simulink model "rtlsdr_QPSK_ascii_message"  (R2021a)
settings: Solver=FixedStepDiscrete  StartTime=0.0  StopTime=60  RelTol=1e-3
PreLoadFcn:
  | %%%%%%%%%%%%%%%%%%%%%%%%%%%%%%%%%%%%%%%%%%%%%%%%%%%%%%%%%%%%%%%%%%%%%%%%%%%
  | % check to see if Simulink library folder is missing from the MATLAB path %
  | %%%%%%%%%%%%%%%%%%%%%%%%%%%%%%%%%%%%%%%%%%%%%%%%%%%%%%%%%%%%%%%%%%%%%%%%%%%
  | if isempty(strfind(path, 'rtlsdr_book_library'))
  | 
  |     % create error window
  |     fig_error = figure(...
  |         'Name', 'Error: RTL-SDR Book Library',...
  |         'Toolbar','none',...
  |         'MenuBar','none',...
  |         'NumberTitle','off',...
  |         'Resize','off',...
  |         'WindowStyle','modal');
  |     fig_error.Position(3) = 600;
  |     fig_error.Position(4) = 150;
  |     fig_axes = axes(...
  |         'Parent',fig_error,...
  |         'Position',[0,0,1,1],...
  |         'visible','off');
  |     % error message
  |     t_title = text(.05,.8,...
  |         'MISSING DIRECTORIES',...
  |         'FontSize',11.5);
  |     t_body = text(.075,.6,...
  |         [{'Simulink cannot find the  \it{<root>}\rm / \it{rtlsdr\_book\_library}\rm  folder in the \it{MATLAB Path}\rm.'},...
  |         {'Please set the MATLAB path following the instructions given in Exercise 2.4.'}],...
  |         'FontSize',10.5);
  |     % buttons
  |     btn_path = uicontrol(...
  |         'Parent',fig_error,...
  |         'String','Set Path Now',...
  |         'FontSize',10,...
  |         'Callback', 'pathtool; close(fig_error);',...
  |         'Position', [fig_error.Position(3)/2-210, 30, 200, 30]);
  |     btn_abort = uicontrol(...
  |         'Parent',fig_error,...
  |         'String','No thanks',...
  |         'FontSize',10,...
  |         'Callback', 'close(fig_error); abort=1;',...
  |         'Position', [fig_error.Position(3)/2+10, 30, 200, 30]);
  | 
  |     % pause to allow user to interact with error box
  |     uiwait(fig_error);
  | 
  |     % abort simulation
  |     try
  |         if abort==1
  |             set_param(gcs, 'SimulationCommand', 'stop');
  |         end
  |     end
  | 
  |     % if user has set path, allow diagram to be updated
  |     if ~exist('abort','var')
  |         % create error window
  |         fig_update = figure(...
  |             'Name', 'Update Diagram',...
  |             'Toolbar','none',...
  |             'MenuBar','none',...
  |             'NumberTitle','off',...
  |             'Resize','off');
  |         fig_update.Position(3) = 400;
  |         fig_update.Position(4) = 120;
  |         fig_axes = axes(...
  |             'Parent',fig_update,...
  |             'Position',[0,0,1,1],...
  |             'visible','off');
  |         % instruction message
  |         t_body = text(.075,.7,...
  |             'Once you have set the path, update the block diagram',...
  |             'FontSize',10.5);
  |         % button
  |         btn_update = uicontrol(...
  |             'Parent',fig_update,...
  |             'String','Update Block Diagram',...
  |             'FontSize',10,...
  |             'Callback', 'set_param(gcs,''SimulationCommand'',''update''); close(gcf)',...
  |             'Position', [fig_update.Position(3)/2-100, 30, 200, 30]);
  |     end
  | 
  |     % clear error components
  |     clear('fig_error','fig_update','fig_axes','t_title','t_body','btn_path','btn_abort','btn_update','abort');
  | 
  | end
  | %%%%%%%%%%%%%%%%%%%%%%%%%%%%%%%%%%%%%%%%%%%%%%%%%%%%%%%%%%%%%%%%%%%%%%%%%%%
  | 
  | 
  | 
  | % ---------------- system parameters ------------------
  | 
  | fs_Tx = 240e3;                           % sampling rate used in the transmitter
  | samp = 50000 - 1;                      % stop time (number of samples in the simulation - 1)
  | fc = 7.5e3;                                  % carrier frequency (IF modulated)
  | Rdata = 2e3;                               % slow data rate chosen for real time demonstration
  | Rsymbol = Rdata/2;                     % QPSK, so 2 samples per symbol
  | fs_Rx = 240e3;                            % sampling rate in the receiver
  | RxDec1 = 5;                                 % decimation at input of Receiver
  | RxDec2 = 6;                                % decimation prior to Coarse Synch
  | RxInt = 3;                                   % interpolation prior to timing and freq synch (output of coarse)
  | OSR = (fs_Rx*RxInt/(RxDec1*RxDec2))/Rsymbol;     % oversampling ratio used in timing and frequency synch
  | 
  | % ---------------- synch loop design ------------------
  | 
  | d = 0.707;                         % damping ratio (using the same for both loops)
  | 
  | % *** CARRIER synch loop *** (note this operates at symbol rate)
  | 
  | T = 1/Rsymbol;                  % sample period
  | Kp = 1;                              % phase detector S-curve is linear
  | Bn = 0.04*Rsymbol;           % bandwidth in Hz
  | Ko = 1;                              % gain of NCO
  | 
  | % calculate the loop filter coefficients for the carrier synch loop
  | K1 = (4*d*Bn*T)/(Ko*Kp*(d+1/(4*d)));
  | K2 = (4*(Bn*T)^2)/(Ko*Kp*(d+1/4*d)^2);
  | 
  | 
  | % *** SYMBOL TIMING synch loop ***
  | 
  | Ts = 1/Rsymbol;                 % symbol period
  | Ks = 3.24;                            % phase detector coefficient
  | BnS = 0.04*Rsymbol;         %  bandwidth in Hz
  | Kn   = 1;                            % gain of numerically controlled clock
  | 
  | % calculate loop filter coefficients
  | Ka = (4*d*BnS*Ts)/(Kn*Ks*(d+1/(4*d)));
  | Kb = (4*(BnS*Ts)^2)/(Kn*Ks*(d+1/4*d)^2);
  | 
  | %------------ design of multirate filter objects ----------
  | 
  | Hd1 = dsp.FIRDecimator(RxDec1,designMultirateFIR(1,RxDec1));            % first stage decimation
  | Hd2 = dsp.FIRDecimator(RxDec2,designMultirateFIR(1,RxDec2));            % second stage decimation
  | Hdf = dsp.FIRDecimator(24,designMultirateFIR(1,24));                           % final stage decimation
  | 
  | Hi = dsp.FIRInterpolator(RxInt,designMultirateFIR(RxInt,1));                   % interpolation
undefined symbols (not defined in the file): rec, src
libraries: simulink_need_slupdate x6, rtlsdr_book_library x5, simulink x4, dspmlti4 x3, dspmtrx3 x3, commdigbbndpm3 x2, commrfcorlib x1, dspbuff3 x1, commutil2 x1, sdrrlib x1, commfilt2 x1
CloseFcn:
  | closefcn_model;
Description:
  | Software, Simulation Examples and Design Exercises Licence Agreement
  | 
  | This license agreement refers to the simulation examples, design exercises and files,
  | and associated software MATLAB and Simulink resources that accompany the book:
  | 
  |      Title: Software Defined Radio using MATLAB & Simulink and the RTL-SDR
  |      Published by Strathclyde Academic Media, 2015
  |      Authored by Robert W. Stewart, Kenneth W. Barlee, Dale S.W. Atkinson,
  |      and Louise H. Crockett
  | 
  | and made available as a download from, www.desktopSDR.com or variously acquired
  | by other means such as via USB storage, cloud storage, disk or any other electronic
  | or optical or magnetic storage mechanism. These files and associated software may
  | be used subject to the terms of agreement of the conditions below:
  | 
  |     Copyright © 2015 Robert W. Stewart, Kenneth W. Barlee, Dale S.W. Atkinson,
  |     and Louise H. Crockett
  |     All rights reserved.
  | 
  | Redistribution and use in source and binary forms, with or without modification, are
  | permitted provided that the following conditions are met:
  | 
  |    1.  Redistributions of source code must retain the above copyright notice, this list of
  |         conditions and the following disclaimer.
  | 
  |    2.  Redistributions in binary form must reproduce the above copyright notice, this
  |         list of conditions and the following disclaimer in the documentation and/or other
  |         materials provided with the distribution.
  | 
  |    3.  Neither the name of the copyright holder nor the names of its contributors may
  |         be used to endorse or promote products derived from this software without
  |         specific prior written permission.
  | 
  |    4.  In all cases, the software is, and all modifications and derivatives of the
  |         software shall be, licensed to you solely for use in conjunction with The
  |         MathWorks, Inc. products and service offerings.
  | 
  | THIS SOFTWARE IS PROVIDED BY THE COPYRIGHT HOLDERS AND CONTRIBUTORS
  | "AS IS" AND ANY EXPRESS OR IMPLIED WARRANTIES, INCLUDING, BUT NOT LIMITED
  | TO, THE IMPLIED WARRANTIES OF MERCHANTABILITY AND FITNESS FOR A
  | PARTICULAR PURPOSE ARE DISCLAIMED. IN NO EVENT SHALL THE COPYRIGHT
  | HOLDER OR CONTRIBUTORS BE LIABLE FOR ANY DIRECT, INDIRECT, INCIDENTAL,
  | SPECIAL, EXEMPLARY, OR CONSEQUENTIAL DAMAGES (INCLUDING, BUT NOT
  | LIMITED TO, PROCUREMENT OF SUBSTITUTE GOODS OR SERVICES; LOSS OF USE,
  | DATA, OR PROFITS; OR BUSINESS INTERRUPTION) HOWEVER CAUSED AND ON ANY
  | THEORY OF LIABILITY, WHETHER IN CONTRACT, STRICT LIABILITY, OR TORT
  | (INCLUDING NEGLIGENCE OR OTHERWISE) ARISING IN ANY WAY OUT OF THE USE
  | OF THIS SOFTWARE, EVEN IF ADVISED OF THE POSSIBILITY OF SUCH DAMAGE.
  | 
  | 
  | Audio Tracks used in Simulations Examples and Design Exercises
  | 
  | The music and vocal files used within the Examples files and software within the book
  | were variously written, arranged, performed, recorded and produced by Garrey Rice,
  | Adam Struth, Jamie Struth, Iain Thistlethwaite and also Marshall Craigmyle who
  | collectively, and individually where appropriate, assert and retain all of their copyright,
  | performance and artistic rights. Permission to use and reproduce this music is
  | granted for all purposes associated with MATLAB and Simulink software and the
  | simulation examples and design exercises files that accompany this book. Requests to
  | use the music for any other purpose should be directed to: info@desktopSDR.com.
  | For information on music track names, full credits, and links to the musicians please
  | refer to www.desktopSDR.com/more/audio.
settings Model: ModifiedByFormat=desktopSDR Team  SimulationMode=accelerator  Creator=desktopSDR Team  LastModifiedBy=desktopSDR Team
settings SolverCC: AlgebraicLoopSolver=TrustRegion
settings DataIOCC: SaveFormat=Array  SaveOutput=off  SignalLogging=off  SaveTime=off  ReturnWorkspaceOutputs=off
settings OptimizationCC: EfficientMapNaN2IntZero=off  LifeSpan=inf
settings DebuggingCC: UnderspecifiedInitializationDetection=Classic  MergeDetectMultiDrivingBlocksExec=none  SolverPrmCheckMsg=warning  ParameterPrecisionLossMsg=none  AllowSymbolicDim=off  SFUnexpectedBacktrackingDiag=warning  SFNoUnconditionalDefaultTransitionDiag=warning  SFExecutionAtInitializationDiag=none  SFMachineParentedDataDiag=warning  ArithmeticOperatorsInVariantConditions=warning
settings HardwareCC: ProdBitPerPointer=32  ProdBitPerSizeT=32  ProdBitPerPtrDiffT=32  ProdLargestAtomicFloat=None  ProdIntDivRoundTo=Undefined  ProdEndianess=Unspecified  ProdWordSize=32  ProdHWDeviceType=32-bit Generic  TargetBitPerPointer=64  TargetBitPerSizeT=64  TargetBitPerPtrDiffT=64  TargetLongLongMode=on  TargetIntDivRoundTo=Zero  TargetEndianess=LittleEndian  TargetWordSize=64  TargetHWDeviceType=MATLAB Host  ProdEqTarget=off
settings ModelReferenceCC: PropagateSignalLabelsOutOfModel=off
settings SFSimCC: SimUseLocalCustomCode=off  CustomCodeUndefinedFunction=UseInterfaceOnly
settings RTWCC: RTWUseLocalCustomCode=off
settings CodeAppCC: MaxIdLength=128  StateflowObjectComments=on
settings GRTTargetCC: TargetLangStandard=C89/C90 (ANSI)  CombineOutputUpdateFcns=off  GRTInterface=on
settings ConfigComp: CovMetricSettings=dw  CovSaveCumulativeToWorkspaceVar=on  CovSaveSingleToWorkspaceVar=on  CovExternalEMLEnable=off  CovSFcnEnable=off

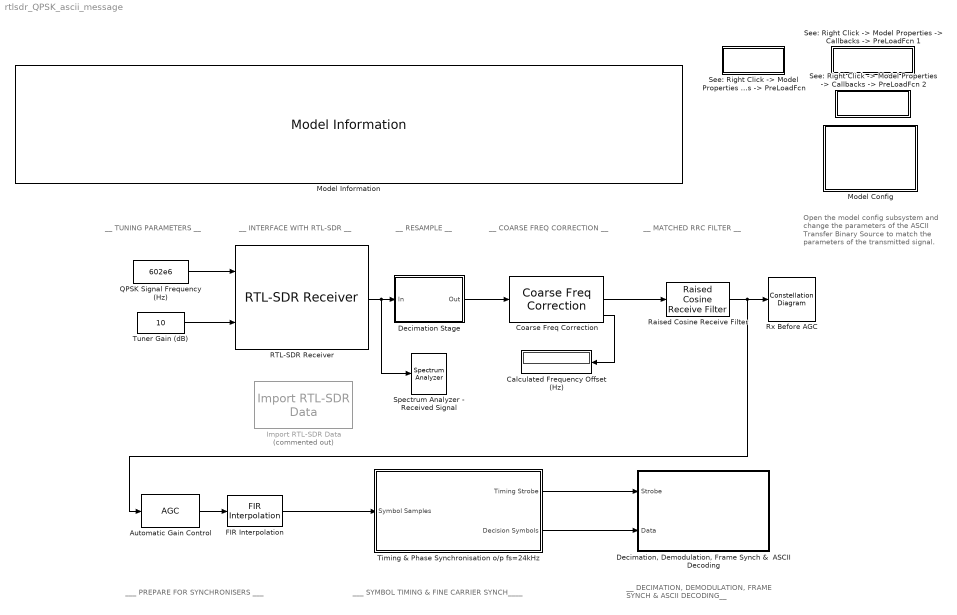
== system rtlsdr_QPSK_ascii_message ==
  note: ___ PREPARE FOR SYNCHRONISERS ___
  note: ___ SYMBOL TIMING & FINE CARRIER SYNCH____
  note: __ DECIMATION, DEMODULATION,
      | FRAME SYNCH & ASCII DECODING__
  note: __ TUNING PARAMETERS __
  note: __ INTERFACE WITH RTL-SDR __
  note: __ RESAMPLE __
  note: __ MATCHED RRC FILTER __
  note: __ COARSE FREQ CORRECTION __
  note: Open the model config subsystem and change the parameters of the ASCII Transfer Binary Source to match the parameters of the transmitted signal.
  Automatic Gain Control : commrfcorlib/AGC  LegacyMode=off  DetectorMethod=Rectifier  LoopMethod=Linear  UpdatePeriod=128  StepSize=0.05  AdaptationStepSize=(0.05)/(128)  DesiredOutputPower=1  AveragingLength=128  MaximumGain=20  MaxPowerGain=20  GainOutputPort=off  InputPowerOutputPort=off  SimulateUsing=Code generation
  Calculated Frequency Offset (Hz) : Display
  Coarse Freq Correction : rtlsdr_book_library/Sync Tools for Digital Comms/Coarse Freq Correction  frm_size=4096
      settings: SourceProductName=RTL-SDR Book Library
  Decimation Stage : Subsystem
      mask Display: disp('Decimation');
  "Decimation, Demodulation, Frame Synch &  ASCII Decoding" : Subsystem  mask(Receiver Parameter Settings){msg_len=rec.msg_len, fs=src.fs, ascii_len=8}
      mask prompts: msg_len "Message Length (chars):"; fs "Sampling Frequency:"; ascii_len "ACSII Length:"
      mask help: This subsystem decimates the signal back to symbol rate by storing only the valid samples that are chosen using the 'strobe' input. It then demodulates the samples back to bits to perform frame synchronisation and finally ASCII decoding. The parameters should match those set in the transmitter for the process to be successful.
      mask Callback msg_len: ASCII_receive_mtchd_filt;
      mask Callback fs: ASCII_receive_mtchd_filt;
      mask Callback ascii_len: ASCII_receive_mtchd_filt;
  FIR Interpolation : dspmlti4/FIR Interpolation  FilterSource=Filter object  PrivateCoeffs=0  h=fir1(71,1/RxInt)  L=RxInt  FilterObject=Hi  InputProcessing=Columns as channels (frame based)  framing=Allow multirate processing  outputBufInitCond=0  roundingMode=Floor  overflowMode=off  firstCoeffDataTypeStr=Inherit: Same word length as input  firstCoeffMin=[]  firstCoeffMax=[]  firstCoeffLastDataTypeStr=Inherit: Same word length as input  outputDataTypeStr=Inherit: Same as accumulator  outputMin=[]  outputMax=[]  outputLastDataTypeStr=Inherit: Same as accumulator
  Import RTL-SDR Data : rtlsdr_book_library/Additional Tools/Import RTL-SDR Data  Commented=on  filename=rec_data\qpsk_ascii_msg.mat  frm_size=4096  data_type=single
      settings: SourceProductName=RTL-SDR Book Library
  Model Config : Subsystem
      mask Display: disp('Model\nConfig')
  Model Information : rtlsdr_book_library/Additional Tools/Model Information/Model Information
      settings: SourceProductName=RTL-SDR Book Library
  "QPSK Signal Frequency (Hz) " : Constant  Value=602e6
  RTL-SDR Receiver : sdrrlib/RTL-SDR Receiver  IPAddress=0  CenterFrequencySource=Input port  CenterFrequency=433.9e6  GainSource=Input port  Gain=15  ADCRate=240e3  FrequencyCorrection=0  LostSamplesOutputPort=off  LatencyOutputPort=off  OutputDataType=single  FrameLength=4096  EnableBurstMode=off  NumFramesInBurst=20  sobjType=sdrr.internal.SDRRTLReceiverSL  dataUDPPort=-1  ctrlUDPPort=-1  subDeviceList=nosubdev  sdrBlockType=SDRBlockTypeSLT.SDRRxBlock  requester=UNUSED_BY_SFCN  sdrExecutionMode=SDRExecutionModeSLT.ExecModeHW  BypassUserLogic=off  DecimatorSelect=DDC decimator  SourceSelect=RF data  SineAmplitude=16000  EnableInternalClock=off  BypassIQBalance=off  IFBandwidth=40e6  ADCRateSource=Dialog  IntermediateFrequency=0  DecimationFactorSource=Dialog  DecimationFactor=512  RFFrequencyIsTunable=logical(1)  SampleTime=(4096)/(240e3)  IFBandwidthSource=Dialog  SineFrequency=30000  BypassDCBlockingFilter=off  IntermediateFrequencySource=Dialog  IQBalanceCoefficients=64  SkipAllHardwareResetAndInitialization=off  EnableIQCalibrationTable=on  CacheIQCalibrationTable=off  EnableOffsetTuning=off  EnableRTLAGC=off  EnableTestMode=off  EnableTunerAGC=off  FrequencyCorrectionSource=Dialog  NumMLBuffers=128  NumUSBBuffers=16  RTLCrystalFrequency=28800000  TunerCrystalFrequency=28800000
      settings: SourceProductBaseCode=RTLSDR
  Raised Cosine Receive Filter : commfilt2/Raised Cosine Receive Filter  filtType=Square root  R=0.5  filtSpan=12  N=fs_Rx/(RxDec1*RxDec2*Rsymbol)  downFactor=1  downOffset=0  filterGain=1  InputProcessing=Columns as channels (frame based)  RateOptions=Enforce single-rate processing  framing=Allow multirate processing  checkCoeff=off  variableName=rcRxFilt1  currentFiltSpan=12  D=(12)/2  inputOffset=0  sampMode=Mute  saveAsFlag=0  rateMode=Downsampling  checkGain=Normalized  launchFVT=on  roundingMode=Floor  overflowMode=off  coeffDataTypeStr=Inherit: Same word length as input  coeffMin=[]  coeffMax=[]  coeffLastDataTypeStr=Inherit: Same word length as input  accumDataTypeStr=Inherit: Same as product output  accumLastDataTypeStr=Inherit: Same as product output  outputDataTypeStr=Inherit: Same as accumulator  outputMin=[]  outputMax=[]  outputLastDataTypeStr=Inherit: Same as accumulator
  Rx Before AGC : ConstellationDiagram
  "See: Right Click -> Model Properties -> Callbacks -> PreLoadFcn" : Subsystem
      mask Display:
      | OSR = evalin('base', 'OSR');
      | fprintf(['OSR = ',num2str(OSR)]);
  "See: Right Click -> Model Properties -> Callbacks -> PreLoadFcn 1" : Subsystem
      mask Display:
      | Rsymbol = evalin('base', 'Rsymbol');
      | fprintf(['Rsymbol = ',num2str(Rsymbol/1e3),' ksps']);
  "See: Right Click -> Model Properties -> Callbacks -> PreLoadFcn 2" : Subsystem
      mask Display:
      | fs_Rx = evalin('base', 'fs_Rx');
      | fprintf(['fs_Rx = ',num2str(fs_Rx/1e3),' kHz']);
  Spectrum Analyzer - Received Signal : SpectrumAnalyzer
  Timing & Phase Synchronisation o/p fs=24kHz : Subsystem
  Tuner Gain (dB) : Constant  Value=10
  wires:
  Raised Cosine Receive Filter/1 -> Rx Before AGC/1, Automatic Gain Control/1
  Automatic Gain Control/1 -> FIR Interpolation/1
  Tuner Gain (dB)/1 -> RTL-SDR Receiver/2
  "QPSK Signal Frequency (Hz) "/1 -> RTL-SDR Receiver/1
  Coarse Freq Correction/2 -> Raised Cosine Receive Filter/1
  FIR Interpolation/1 -> Timing & Phase Synchronisation o/p fs=24kHz/1(Symbol Samples)
  Timing & Phase Synchronisation o/p fs=24kHz/2(Decision Symbols) -> "Decimation, Demodulation, Frame Synch &  ASCII Decoding"/2(Data)
  Decimation Stage/1(Out) -> Coarse Freq Correction/1
  Coarse Freq Correction/3 -> Calculated Frequency Offset (Hz)/1
  Timing & Phase Synchronisation o/p fs=24kHz/1(Timing Strobe) -> "Decimation, Demodulation, Frame Synch &  ASCII Decoding"/1(Strobe)
  RTL-SDR Receiver/1 -> Spectrum Analyzer - Received Signal/1, Decimation Stage/1(In)

== system rtlsdr_QPSK_ascii_message/Decimation Stage ==
  In : Inport
  FIR Decimation x5 o/p fs=48kHz : dspmlti4/FIR Decimation  FilterSource=Filter object  h=fir1(35,1/5)  D=5  filtStruct=Direct form  FilterObject=Hd1  InputProcessing=Columns as channels (frame based)  framing=Allow multirate processing  inputOffset=0  outputBufInitCond=0  roundingMode=Floor  overflowMode=off  firstCoeffDataTypeStr=Inherit: Same word length as input  firstCoeffMin=[]  firstCoeffMax=[]  firstCoeffLastDataTypeStr=Inherit: Same word length as input  outputDataTypeStr=Inherit: Same as accumulator  outputMin=[]  outputMax=[]  outputLastDataTypeStr=Inherit: Same as accumulator
  "FIR Decimation x6 o/p fs=8kHz " : dspmlti4/FIR Decimation  FilterSource=Filter object  h=fir1(75,1/6)  D=6  filtStruct=Direct form  FilterObject=Hd2  InputProcessing=Columns as channels (frame based)  framing=Allow multirate processing  inputOffset=0  outputBufInitCond=0  roundingMode=Floor  overflowMode=off  firstCoeffDataTypeStr=Inherit: Same word length as input  firstCoeffMin=[]  firstCoeffMax=[]  firstCoeffLastDataTypeStr=Inherit: Same word length as input  outputDataTypeStr=Inherit: Same as accumulator  outputMin=[]  outputMax=[]  outputLastDataTypeStr=Inherit: Same as accumulator
  Out : Outport
  wires:
  "FIR Decimation x6 o/p fs=8kHz "/1 -> Out/1
  FIR Decimation x5 o/p fs=48kHz/1 -> "FIR Decimation x6 o/p fs=8kHz "/1
  In/1 -> FIR Decimation x5 o/p fs=48kHz/1

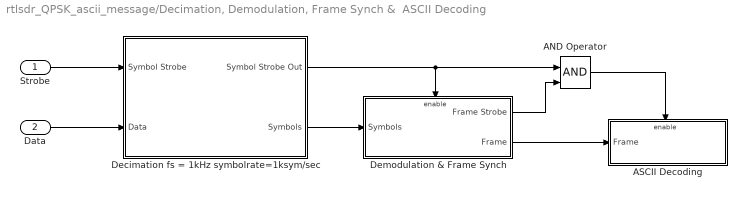
== system rtlsdr_QPSK_ascii_message/Decimation, Demodulation, Frame Synch &  ASCII Decoding ==
  Strobe : Inport
  Data : Inport  Port=2
  AND Operator : Logic  IconShape=distinctive  AllPortsSameDT=off  OutDataTypeStr=boolean
  ASCII Decoding : Subsystem
  Decimation fs = 1kHz symbolrate=1ksym/sec : Subsystem
  Demodulation & Frame Synch : Subsystem
  wires:
  Strobe/1 -> Decimation fs = 1kHz symbolrate=1ksym/sec/1(Symbol Strobe)
  Data/1 -> Decimation fs = 1kHz symbolrate=1ksym/sec/2(Data)
  Decimation fs = 1kHz symbolrate=1ksym/sec/2(Symbols) -> Demodulation & Frame Synch/1(Symbols)
  Decimation fs = 1kHz symbolrate=1ksym/sec/1(Symbol Strobe Out) -> AND Operator/1, Demodulation & Frame Synch/Enable
  Demodulation & Frame Synch/2(Frame) -> ASCII Decoding/1(Frame)
  AND Operator/1 -> ASCII Decoding/Enable
  Demodulation & Frame Synch/1(Frame Strobe) -> AND Operator/2

== system rtlsdr_QPSK_ascii_message/Model Config ==
  "  ASCII Transfer Binary Source" : rtlsdr_book_library/Data Comms Sources and Sinks/  ASCII Transfer Binary Source  msg_tx=Hello World!  fs=2e3
      settings: SourceProductName=RTL-SDR Book Library
  Terminator : Terminator
  wires:
  "  ASCII Transfer Binary Source"/1 -> Terminator/1

== system rtlsdr_QPSK_ascii_message/See: Right Click -> Model Properties -> Callbacks -> PreLoadFcn ==

== system rtlsdr_QPSK_ascii_message/See: Right Click -> Model Properties -> Callbacks -> PreLoadFcn 1 ==

== system rtlsdr_QPSK_ascii_message/See: Right Click -> Model Properties -> Callbacks -> PreLoadFcn 2 ==

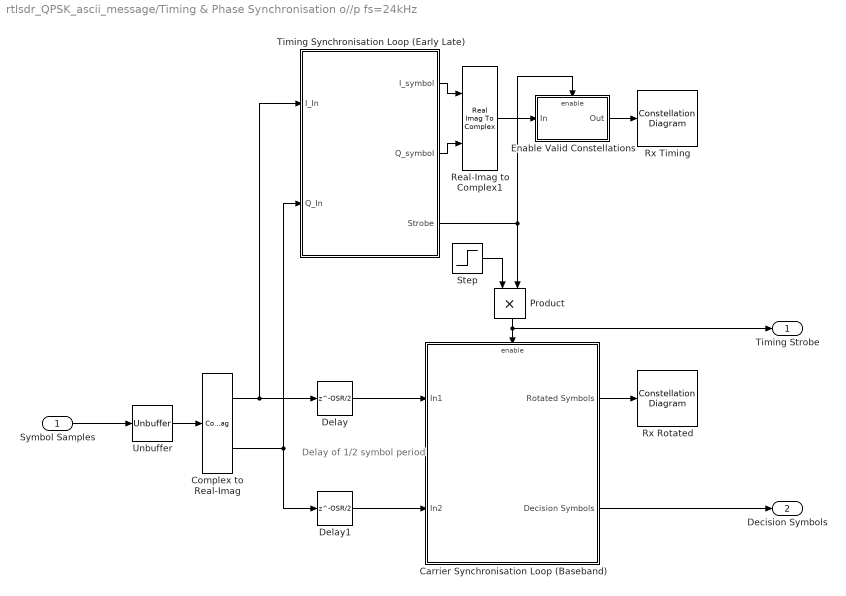
== system rtlsdr_QPSK_ascii_message/Timing & Phase Synchronisation o//p fs=24kHz ==
  note: Delay of 1/2
      | symbol period
  Symbol Samples : Inport
  Carrier Synchronisation Loop (Baseband) : Subsystem
  Complex to Real-Imag : ComplexToRealImag
  Delay : Delay  DelayLength=OSR/2  InitialCondition=1.0
  Delay1 : Delay  DelayLength=OSR/2  InitialCondition=1.0
  Enable Valid Constellations : Subsystem  TreatAsAtomicUnit=on
  Product : Product
  Real-Imag to Complex1 : RealImagToComplex
  Rx Rotated : ConstellationDiagram
  Rx Timing : ConstellationDiagram
  Step : Step  Time=0.75  SampleTime=(RxDec1*RxDec2)/(fs_Rx*RxInt)
  Timing Synchronisation Loop (Early Late) : Subsystem  mask(Early Late Timing Error Detector){OSR=OSR, Ka=Ka, Kb=Kb}
      mask prompts: OSR "Oversampling ratio (even integer value)"; Ka "Ka (Loop Filter proportial gain)"; Kb "Kb (Loop Filter integral gain)"
      mask help:
      | This TED works with quadrature (I and Q) inputs and generates a strobe for sampling the punctual branch at the optimal timing instants.
      |
      | The model can be parameterised in terms of the oversampling ratio and the design of the timing PLL.
      |
      | Note that the oversampling ratio must be an EVEN INTEGER value.
  Unbuffer : Unbuffer  ic=0.7071+0.7071i
  Timing Strobe : Outport
  Decision Symbols : Outport  Port=2
  wires:
  Timing Synchronisation Loop (Early Late)/1(I_symbol) -> Real-Imag to Complex1/1
  Delay/1 -> Carrier Synchronisation Loop (Baseband)/1(In1)
  Delay1/1 -> Carrier Synchronisation Loop (Baseband)/2(In2)
  Product/1 -> Carrier Synchronisation Loop (Baseband)/Enable, Timing Strobe/1
  Carrier Synchronisation Loop (Baseband)/1(Rotated Symbols) -> Rx Rotated/1
  Complex to Real-Imag/1 -> Delay/1, Timing Synchronisation Loop (Early Late)/1(I_In)
  Complex to Real-Imag/2 -> Delay1/1, Timing Synchronisation Loop (Early Late)/2(Q_In)
  Enable Valid Constellations/1(Out) -> Rx Timing/1
  Carrier Synchronisation Loop (Baseband)/2("Decision Symbols ") -> Decision Symbols/1
  Timing Synchronisation Loop (Early Late)/3(Strobe) -> Product/2, Enable Valid Constellations/Enable
  Real-Imag to Complex1/1 -> Enable Valid Constellations/1(In)
  Timing Synchronisation Loop (Early Late)/2(Q_symbol) -> Real-Imag to Complex1/2
  Step/1 -> Product/1
  Symbol Samples/1 -> Unbuffer/1
  Unbuffer/1 -> Complex to Real-Imag/1

== system rtlsdr_QPSK_ascii_message/Decimation, Demodulation, Frame Synch &  ASCII Decoding/ASCII Decoding ==
  Frame : Inport
  Enable : EnablePort
  ASCII Decoding : rtlsdr_book_library/Data Comms Sources and Sinks/ASCII Decoding  msg_len=rec.msg_len  ascii_len=rec.ascii_len
      settings: SourceProductName=RTL-SDR Book Library
  Remove Preamble : dspmtrx3/Submatrix  RowSpan=Range of rows  RowStartMode=Index  RowStartIndex=rec.preamble_len+rec.preamble_pad_len+1  RowEndMode=Index  RowEndIndex=rec.master_frame_len-rec.frame_pad_len  ColSpan=One column  ColStartMode=First  ColStartIndex=1  ColEndMode=Last  ColEndIndex=1
  wires:
  Frame/1 -> Remove Preamble/1
  Remove Preamble/1 -> ASCII Decoding/1

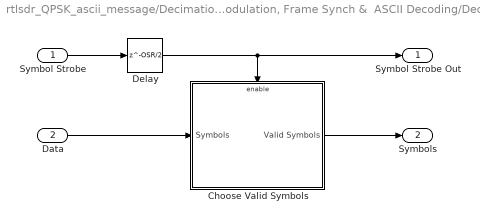
== system rtlsdr_QPSK_ascii_message/Decimation, Demodulation, Frame Synch &  ASCII Decoding/Decimation fs = 1kHz symbolrate=1ksym//sec ==
  Symbol Strobe : Inport
  Data : Inport  Port=2
  Choose Valid Symbols : Subsystem
  Delay : Delay  DelayLength=OSR/2  InitialCondition=1
  Symbol Strobe Out : Outport
  Symbols : Outport  Port=2
  wires:
  Symbol Strobe/1 -> Delay/1
  Data/1 -> Choose Valid Symbols/1(Symbols)
  Delay/1 -> Choose Valid Symbols/Enable, Symbol Strobe Out/1
  Choose Valid Symbols/1(Valid Symbols) -> Symbols/1

== system rtlsdr_QPSK_ascii_message/Decimation, Demodulation, Frame Synch &  ASCII Decoding/Demodulation & Frame Synch ==
  Symbols : Inport
  Enable : EnablePort
  Demodulation & Phase Ambiguity Correction : Subsystem
  Frame Synchronisation : Subsystem
  Frame Strobe : Outport
  Frame : Outport  Port=2
  wires:
  Symbols/1 -> Demodulation & Phase Ambiguity Correction/1(Data)
  Demodulation & Phase Ambiguity Correction/1(Corrected Data) -> Frame Synchronisation/1(Bit Pairs)
  Frame Synchronisation/1(Frame) -> Frame/1
  Frame Synchronisation/2(Frame Strobe) -> Frame Strobe/1

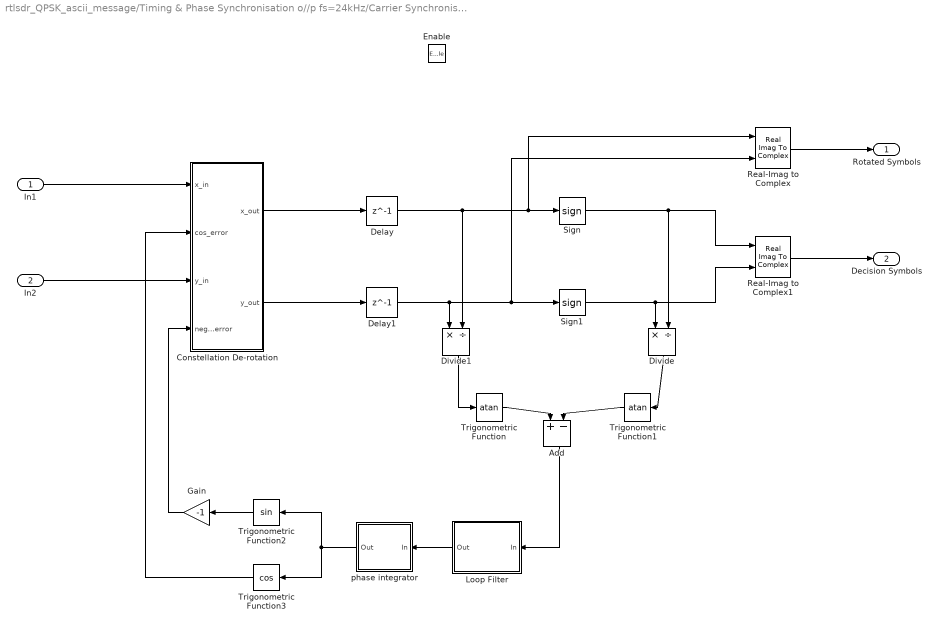
== system rtlsdr_QPSK_ascii_message/Timing & Phase Synchronisation o//p fs=24kHz/Carrier Synchronisation Loop (Baseband) ==
  In1 : Inport
  In2 : Inport  Port=2
  Enable : EnablePort
  Add : Sum  Inputs=+-
  Constellation De-rotation : Subsystem
  Delay : Delay  DelayLength=1  InitialCondition=1
  Delay1 : Delay  DelayLength=1  InitialCondition=0
  Divide : Product  Inputs=*/
  Divide1 : Product  Inputs=*/
  Gain : Gain  Gain=-1
  Loop Filter : Subsystem
  Real-Imag to Complex : RealImagToComplex
  Real-Imag to Complex1 : RealImagToComplex
  Sign : Signum
  Sign1 : Signum
  Trigonometric Function : Trigonometry  Operator=atan  OutputSignalType=real
  Trigonometric Function1 : Trigonometry  Operator=atan  OutputSignalType=real
  Trigonometric Function2 : Trigonometry
  Trigonometric Function3 : Trigonometry  Operator=cos
  phase integrator : Subsystem
  Rotated Symbols : Outport
  "Decision Symbols " : Outport  Port=2
  wires:
  Sign/1 -> Divide/2, Real-Imag to Complex1/1
  Sign1/1 -> Divide/1, Real-Imag to Complex1/2
  Trigonometric Function/1 -> Add/1
  Trigonometric Function1/1 -> Add/2
  Divide/1 -> Trigonometric Function1/1
  Divide1/1 -> Trigonometric Function/1
  Gain/1 -> Constellation De-rotation/4(neg_sin_error)
  Delay/1 -> Divide1/2, Real-Imag to Complex/1, Sign/1
  Delay1/1 -> Divide1/1, Sign1/1, Real-Imag to Complex/2
  Real-Imag to Complex1/1 -> "Decision Symbols "/1
  Trigonometric Function2/1 -> Gain/1
  Constellation De-rotation/1(x_out) -> Delay/1
  Loop Filter/1(Out) -> phase integrator/1(In)
  Constellation De-rotation/2(y_out) -> Delay1/1
  In1/1 -> Constellation De-rotation/1(x_in)
  In2/1 -> Constellation De-rotation/3(y_in)
  Add/1 -> Loop Filter/1(In)
  phase integrator/1(Out) -> Trigonometric Function2/1, Trigonometric Function3/1
  Trigonometric Function3/1 -> Constellation De-rotation/2(cos_error)
  Real-Imag to Complex/1 -> Rotated Symbols/1

== system rtlsdr_QPSK_ascii_message/Timing & Phase Synchronisation o//p fs=24kHz/Enable Valid Constellations ==
  In : Inport
  Enable : EnablePort
  Out : Outport
  wires:
  In/1 -> Out/1

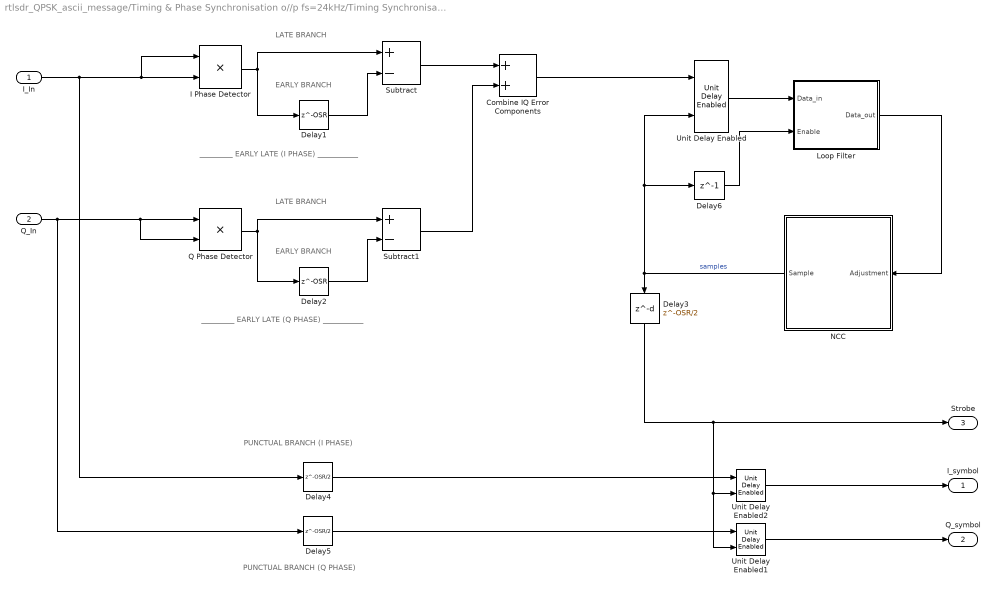
== system rtlsdr_QPSK_ascii_message/Timing & Phase Synchronisation o//p fs=24kHz/Timing Synchronisation Loop (Early Late) ==
  note: LATE BRANCH
  note: EARLY BRANCH
  note: LATE BRANCH
  note: EARLY BRANCH
  note: _________ EARLY LATE (I PHASE) ___________
  note: _________ EARLY LATE (Q PHASE) ___________
  note: PUNCTUAL BRANCH (I PHASE)
  note: PUNCTUAL BRANCH (Q PHASE)
  I_In : Inport
  Q_In : Inport  Port=2
  Combine IQ Error Components : Sum
  Delay1 : Delay  DelayLength=OSR
  Delay2 : Delay  DelayLength=OSR
  Delay3 : Delay  DelayLength=OSR/2
  Delay4 : Delay  DelayLength=OSR/2  InitialCondition=1.0
  Delay5 : Delay  DelayLength=OSR/2  InitialCondition=1.0
  Delay6 : Delay  DelayLength=1
  I Phase Detector : Product
  Loop Filter : Subsystem
  NCC : Subsystem  mask(Numerically Controller Clock (NCC)){OSR=OSR}
      mask prompts: OSR "Oversampling Ratio"
      mask help:
      | This component operates similarly to a Numerically Controlled Oscillator (NCO).
      |
      | Internally, a nominal step size of (1 + Adjustment) is applied to an accumulator. The accumulator wraps around at N = OSR, therefore for a zero control input, the accumulator wraps once every symbol period at the expected rate.
      |
      | When the accumulator wraps, a strobe output is produced.
  Q Phase Detector : Product
  Subtract : Sum  Inputs=+-
  Subtract1 : Sum  Inputs=+-
  Unit Delay Enabled : simulink_need_slupdate/Unit Delay Enabled  vinit=0.0  tsamp=-1
      settings: SourceProductBaseCode=SL
  Unit Delay Enabled1 : simulink_need_slupdate/Unit Delay Enabled  vinit=0.0  tsamp=-1
      settings: SourceProductBaseCode=SL
  Unit Delay Enabled2 : simulink_need_slupdate/Unit Delay Enabled  vinit=0.0  tsamp=-1
      settings: SourceProductBaseCode=SL
  I_symbol : Outport
  Q_symbol : Outport  Port=2
  Strobe : Outport  Port=3
  wires:
  Delay2/1 -> Subtract1/2
  Subtract1/1 -> Combine IQ Error Components/2
  Unit Delay Enabled/1 -> Loop Filter/1(Data_in)
  Combine IQ Error Components/1 -> Unit Delay Enabled/1
  I Phase Detector/1 -> Subtract/1, Delay1/1
  Delay1/1 -> Subtract/2
  NCC/1(Sample) -> Unit Delay Enabled/2, Delay6/1, Delay3/1  "samples"
  Subtract/1 -> Combine IQ Error Components/1
  Q Phase Detector/1 -> Delay2/1, Subtract1/1
  Loop Filter/1(Data_out) -> NCC/1(Adjustment)
  Delay6/1 -> Loop Filter/2(Enable)
  Q_In/1 -> Delay5/1, Q Phase Detector/2, Q Phase Detector/1
  I_In/1 -> Delay4/1, I Phase Detector/1, I Phase Detector/2
  Delay4/1 -> Unit Delay Enabled2/1
  Delay5/1 -> Unit Delay Enabled1/1
  Delay3/1 -> Strobe/1, Unit Delay Enabled1/2, Unit Delay Enabled2/2
  Unit Delay Enabled2/1 -> I_symbol/1
  Unit Delay Enabled1/1 -> Q_symbol/1

== system rtlsdr_QPSK_ascii_message/Decimation, Demodulation, Frame Synch &  ASCII Decoding/Decimation fs = 1kHz symbolrate=1ksym//sec/Choose Valid Symbols ==
  Symbols : Inport
  Enable : EnablePort
  Valid Symbols : Outport
  wires:
  Symbols/1 -> Valid Symbols/1

== system rtlsdr_QPSK_ascii_message/Decimation, Demodulation, Frame Synch &  ASCII Decoding/Demodulation & Frame Synch/Demodulation & Phase Ambiguity Correction ==
  Data : Inport
  DQPSK Demodulator Baseband : commdigbbndpm3/DQPSK Demodulator Baseband  OutType=Bit  Dec=Gray  Ph=pi/2  outDtype1=single  outDtype2=Inherit via internal rule
      settings: SourceProductBaseCode=CM
  Manual Switch : ManualSwitch
  QPSK Demodulator Baseband : commdigbbndpm3/QPSK Demodulator Baseband  OutType=Bit  DecType=Hard decision  VarSource=Dialog  Variance=1  Dec=Gray  Ph=pi/4  outDtype1=single  outDtype2=Inherit via internal rule  derotateFactorWordLen=16  derotateFactorDataTypeStr=Inherit: Same word length as input  derotateFactorLastDataTypeStr=Inherit: Same word length as input
  Corrected Data : Outport
  wires:
  DQPSK Demodulator Baseband/1 -> Manual Switch/2
  QPSK Demodulator Baseband/1 -> Manual Switch/1
  Manual Switch/1 -> Corrected Data/1
  Data/1 -> DQPSK Demodulator Baseband/1, QPSK Demodulator Baseband/1

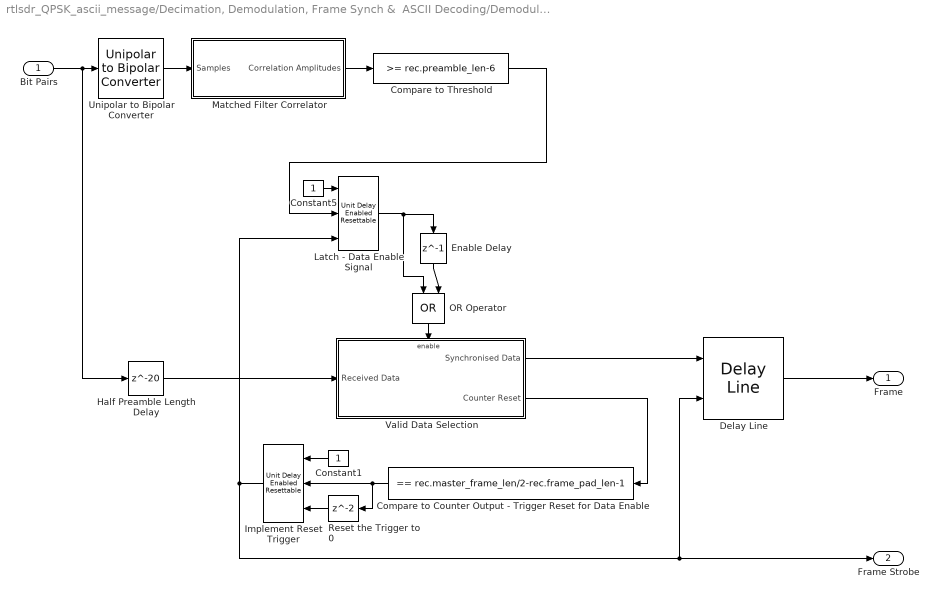
== system rtlsdr_QPSK_ascii_message/Decimation, Demodulation, Frame Synch &  ASCII Decoding/Demodulation & Frame Synch/Frame Synchronisation ==
  Bit Pairs : Inport
  Compare to Counter Output - Trigger Reset for Data Enable : simulink/Logic and Bit Operations/Compare To Constant  relop===  const=rec.master_frame_len/2-rec.frame_pad_len-1  OutDataTypeStr=boolean
  Compare to Threshold : simulink/Logic and Bit Operations/Compare To Constant  relop=>=  const=rec.preamble_len-6  OutDataTypeStr=boolean
  Constant1 : Constant  OutDataTypeStr=boolean
  Constant5 : Constant
  Delay Line : dspbuff3/Delay Line  siz=rec.master_frame_len-rec.frame_pad_len  ic=0  directfeed=on  enable_output=on  hold_output=off  OutputFrames=on
      settings: SourceProductBaseCode=DS
  Enable Delay : Delay  DelayLength=1  InitialCondition=0
  Half Preamble Length Delay : Delay  DelayLength=20  InitialCondition=0
  Implement Reset Trigger : simulink_need_slupdate/Unit Delay Enabled Resettable  vinit=0  tsamp=-1
      settings: SourceProductBaseCode=SL
  Latch - Data Enable Signal : simulink_need_slupdate/Unit Delay Enabled Resettable  vinit=0  tsamp=-1
      settings: SourceProductBaseCode=SL
  Matched Filter Correlator : Subsystem
  OR Operator : Logic  Operator=OR  IconShape=distinctive  AllPortsSameDT=off  OutDataTypeStr=boolean
  Reset the Trigger to 0 : Delay  DelayLengthUpperLimit=10000  InitialCondition=0
  Unipolar to Bipolar Converter : commutil2/Unipolar to Bipolar Converter  M=2  polarity=Positive  dataType=Inherit via internal rule
  Valid Data Selection : Subsystem
  Frame : Outport
  Frame Strobe : Outport  Port=2
  wires:
  Compare to Counter Output - Trigger Reset for Data Enable/1 -> Reset the Trigger to 0/1, Implement Reset Trigger/2
  Matched Filter Correlator/1(Correlation Amplitudes) -> Compare to Threshold/1
  Latch - Data Enable Signal/1 -> Enable Delay/1, OR Operator/1
  Valid Data Selection/2(Counter Reset) -> Compare to Counter Output - Trigger Reset for Data Enable/1
  Valid Data Selection/1(Synchronised Data) -> Delay Line/1
  Enable Delay/1 -> OR Operator/2
  Constant1/1 -> Implement Reset Trigger/1
  Delay Line/1 -> Frame/1
  Implement Reset Trigger/1 -> Frame Strobe/1, Delay Line/2, Latch - Data Enable Signal/3
  Unipolar to Bipolar Converter/1 -> Matched Filter Correlator/1(Samples)
  Half Preamble Length Delay/1 -> Valid Data Selection/1(Received Data)
  Bit Pairs/1 -> Unipolar to Bipolar Converter/1, Half Preamble Length Delay/1
  Compare to Threshold/1 -> Latch - Data Enable Signal/2
  Reset the Trigger to 0/1 -> Implement Reset Trigger/3
  Constant5/1 -> Latch - Data Enable Signal/1
  OR Operator/1 -> Valid Data Selection/Enable

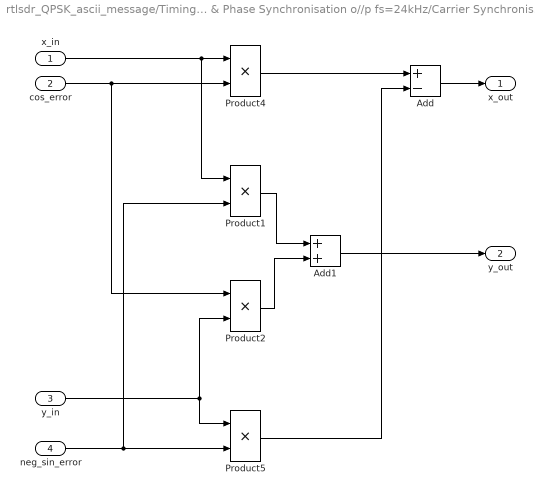
== system rtlsdr_QPSK_ascii_message/Timing & Phase Synchronisation o//p fs=24kHz/Carrier Synchronisation Loop (Baseband)/Constellation De-rotation ==
  x_in : Inport
  cos_error : Inport  Port=2
  y_in : Inport  Port=3
  neg_sin_error : Inport  Port=4
  Add : Sum  Inputs=+-
  Add1 : Sum
  Product{1..2,4..5} (4 alike) : Product
  x_out : Outport
  y_out : Outport  Port=2
  wires:
  Product4/1 -> Add/1
  Product5/1 -> Add/2
  cos_error/1 -> Product2/1, Product4/2
  Add/1 -> x_out/1
  neg_sin_error/1 -> Product5/2, Product1/2
  Product2/1 -> Add1/2
  Product1/1 -> Add1/1
  Add1/1 -> y_out/1
  y_in/1 -> Product5/1, Product2/2
  x_in/1 -> Product4/1, Product1/1

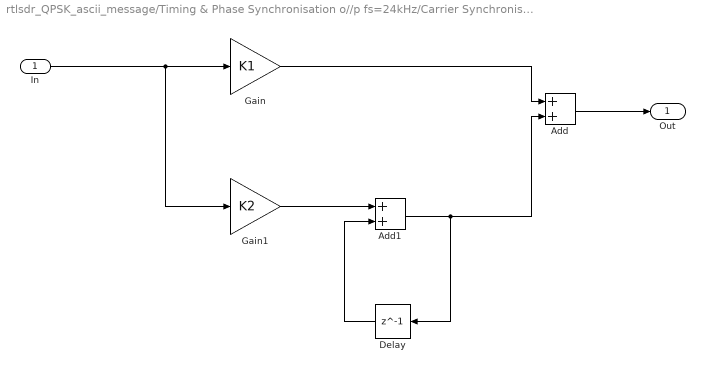
== system rtlsdr_QPSK_ascii_message/Timing & Phase Synchronisation o//p fs=24kHz/Carrier Synchronisation Loop (Baseband)/Loop Filter ==
  In : Inport
  Add : Sum
  Add1 : Sum
  Delay : Delay  DelayLength=1  InitialCondition=0
  Gain : Gain  Gain=K1
  Gain1 : Gain  Gain=K2
  Out : Outport
  wires:
  Gain1/1 -> Add1/1
  Add/1 -> Out/1
  Gain/1 -> Add/1
  Delay/1 -> Add1/2
  Add1/1 -> Delay/1, Add/2
  In/1 -> Gain1/1, Gain/1

== system rtlsdr_QPSK_ascii_message/Timing & Phase Synchronisation o//p fs=24kHz/Carrier Synchronisation Loop (Baseband)/phase integrator ==
  In : Inport
  Add : Sum
  Delay : Delay  DelayLength=1  InitialCondition=0
  Gain : Gain  Gain=Ko
  Out : Outport
  wires:
  In/1 -> Add/1
  Add/1 -> Delay/1, Gain/1
  Delay/1 -> Add/2
  Gain/1 -> Out/1

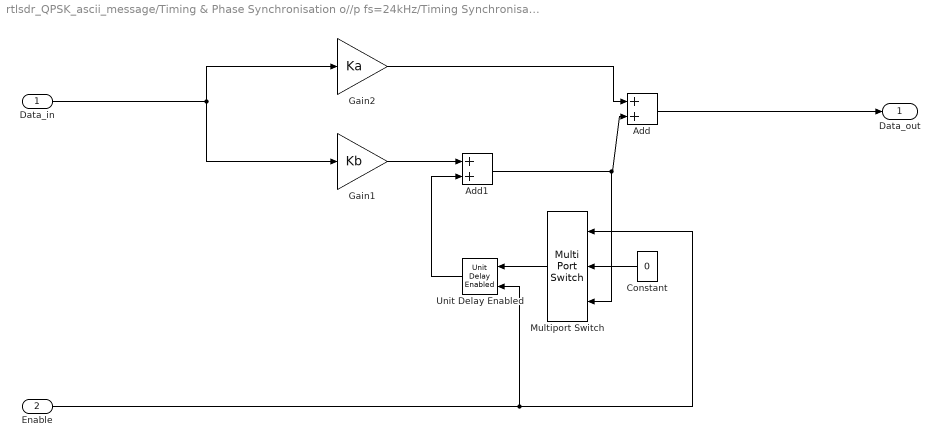
== system rtlsdr_QPSK_ascii_message/Timing & Phase Synchronisation o//p fs=24kHz/Timing Synchronisation Loop (Early Late)/Loop Filter ==
  Data_in : Inport
  Enable : Inport  Port=2
  Add : Sum
  Add1 : Sum
  Constant : Constant  Value=0  SampleTime=(RxDec1*RxDec2)/(fs_Rx*RxInt)
  Gain1 : Gain  Gain=Kb
  Gain2 : Gain  Gain=Ka
  Multiport Switch : MultiPortSwitch  DataPortOrder=Zero-based contiguous  Inputs=2  zeroidx=on
  Unit Delay Enabled : simulink_need_slupdate/Unit Delay Enabled  vinit=0.0  tsamp=-1
      settings: SourceProductBaseCode=SL
  Data_out : Outport
  wires:
  Gain1/1 -> Add1/1
  Gain2/1 -> Add/1
  Unit Delay Enabled/1 -> Add1/2
  Add1/1 -> Multiport Switch/3, Add/2
  Data_in/1 -> Gain2/1, Gain1/1
  Add/1 -> Data_out/1
  Enable/1 -> Unit Delay Enabled/2, Multiport Switch/1
  Multiport Switch/1 -> Unit Delay Enabled/1
  Constant/1 -> Multiport Switch/2

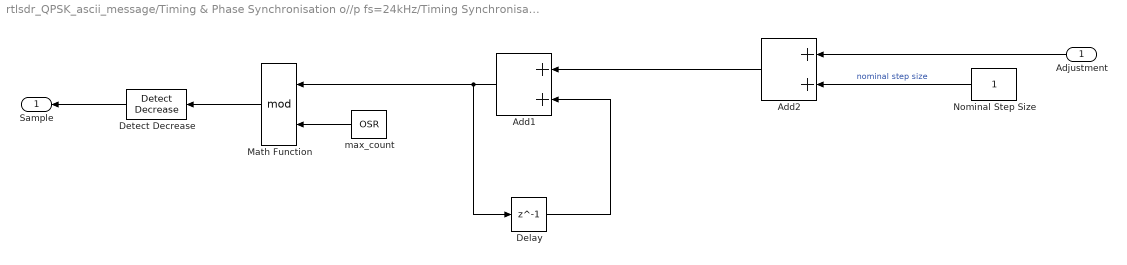
== system rtlsdr_QPSK_ascii_message/Timing & Phase Synchronisation o//p fs=24kHz/Timing Synchronisation Loop (Early Late)/NCC ==
  Adjustment : Inport
  Add1 : Sum  OutDataTypeStr=double
  Add2 : Sum  OutDataTypeStr=double
  Delay : Delay  DelayLength=1
  Detect Decrease : simulink/Logic and Bit Operations/Detect Decrease  vinit=0.0  OutDataTypeStr=boolean
  Math Function : Math  Operator=mod  SignedPower=on  SaturateOnIntegerOverflow=on
  Nominal Step Size : Constant  OutDataTypeStr=double  SampleTime=(RxDec1*RxDec2)/(fs_Rx*RxInt)
  max_count : Constant  Value=OSR  OutDataTypeStr=double  SampleTime=(RxDec1*RxDec2)/(fs_Rx*RxInt)
  Sample : Outport
  wires:
  Adjustment/1 -> Add2/1
  Add2/1 -> Add1/1
  Delay/1 -> Add1/2
  Nominal Step Size/1 -> Add2/2  "nominal step size"
  Add1/1 -> Delay/1, Math Function/1
  Math Function/1 -> Detect Decrease/1
  max_count/1 -> Math Function/2
  Detect Decrease/1 -> Sample/1

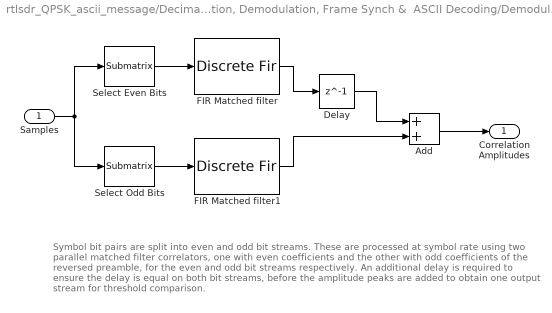
== system rtlsdr_QPSK_ascii_message/Decimation, Demodulation, Frame Synch &  ASCII Decoding/Demodulation & Frame Synch/Frame Synchronisation/Matched Filter Correlator ==
  note: Symbol bit pairs are split into even and odd bit streams. These are processed at symbol rate using
      | two parallel matched filter correlators, one with even coefficients and the other with odd coefficients
      | of the reversed preamble, for the even and odd bit streams respectively. An additional delay is
      | required to ensure the delay is equal on both bit streams, before the amplitude peaks are added to
      | obtain one output stream for threshold comparison.
  Samples : Inport
  Add : Sum
  Delay : Delay  DelayLength=1  InitialCondition=0
  FIR Matched filter : DiscreteFir  Coefficients=rec.filter_coeff_even
  FIR Matched filter1 : DiscreteFir  Coefficients=rec.filter_coeff_odd
  Select Even Bits : dspmtrx3/Submatrix  RowSpan=One row  RowStartMode=Index  RowStartIndex=2  RowEndMode=Index  RowEndIndex=1  ColSpan=One column  ColStartMode=Index  ColStartIndex=1  ColEndMode=Last  ColEndIndex=1
  Select Odd Bits : dspmtrx3/Submatrix  RowSpan=One row  RowStartMode=Index  RowStartIndex=1  RowEndMode=Index  RowEndIndex=rec.master_frame_len-rec.pad  ColSpan=One column  ColStartMode=Index  ColStartIndex=1  ColEndMode=Last  ColEndIndex=1
  Correlation Amplitudes : Outport
  wires:
  Select Odd Bits/1 -> FIR Matched filter1/1
  Samples/1 -> Select Odd Bits/1, Select Even Bits/1
  FIR Matched filter1/1 -> Add/2
  Delay/1 -> Add/1
  Select Even Bits/1 -> FIR Matched filter/1
  FIR Matched filter/1 -> Delay/1
  Add/1 -> Correlation Amplitudes/1

== system rtlsdr_QPSK_ascii_message/Decimation, Demodulation, Frame Synch &  ASCII Decoding/Demodulation & Frame Synch/Frame Synchronisation/Valid Data Selection ==
  Received Data : Inport
  Enable : EnablePort
  Counter Limited : simulink/Sources/Counter Limited  uplimit=rec.master_frame_len/2-rec.frame_pad_len  tsamp=-1
  Reshape : Reshape
  Synchronised Data : Outport
  Counter Reset : Outport  Port=2  InitialOutput=0
  wires:
  Counter Limited/1 -> Counter Reset/1
  Received Data/1 -> Reshape/1
  Reshape/1 -> Synchronised Data/1
